simulink model "OSWT"  (R2022a)
settings: Solver=ode5  StartTime=0.0  StopTime=inf  RelTol=1e-3
model workspace (MAT data in the model file):
  autoELoad = 0
  autoPitch = 0
  eLoad = 0
  pitch = 0
libraries: simulink x1, sldrtlib x1
settings Model: SimulationMode=external  Creator=segu222  LastModifiedBy=belensanchezcenteno
settings DataIOCC: ReturnWorkspaceOutputs=off
settings DebuggingCC: UnconnectedInputMsg=warning  UnconnectedOutputMsg=warning  UnconnectedLineMsg=warning
settings HardwareCC: ProdBitPerLong=64  ProdHWDeviceType=Intel->x86-64 (Linux 64)
settings RTWCC: Description=Simulink Desktop Real-Time  SystemTargetFile=sldrt.tlc  TemplateMakefile=sldrt.tmf  RTWCompilerOptimization=on  DLArmComputeVersion=19.05
settings CodeAppCC: MaxIdLength=95
settings SimulinkDesktopRealTimeCC: TargetLibSuffix=_sldrt.a  TargetPreCompLibLocation=/Applications/MATLAB_R2022a.app/toolbox/sldrt/lib/maci64

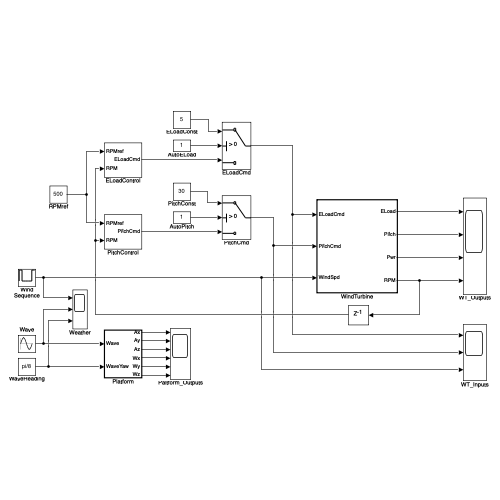
[thumbnail: Simulink's stored preview of the top-level diagram]
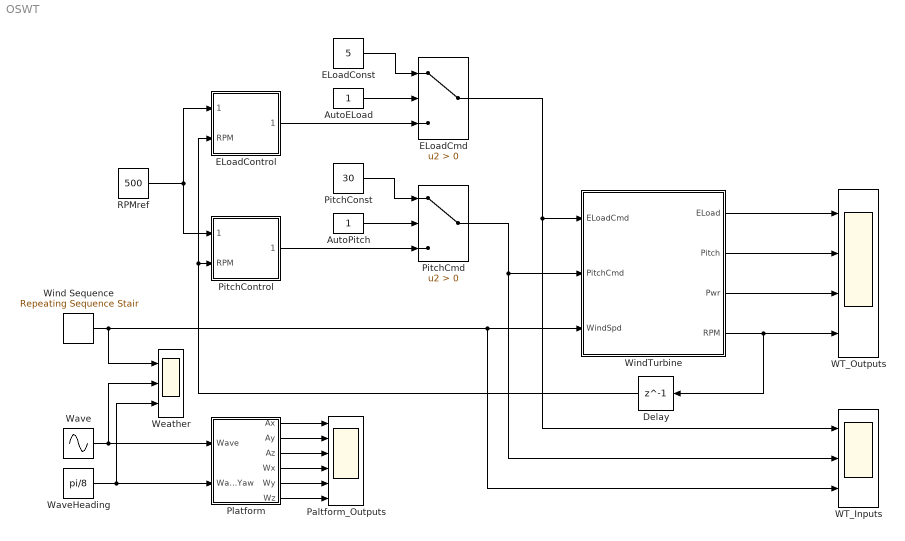
== system OSWT ==
  AutoELoad : Constant
  AutoPitch : Constant  VectorParams1D=off
  Delay : Delay  DelayLength=1
  ELoadCmd : Switch  Criteria=u2 > Threshold  SaturateOnIntegerOverflow=off  InputSameDT=off
  ELoadConst : Constant  Value=5
  ELoadControl : Subsystem
  Paltform_Outputs : Scope  NumInputPorts=6
  PitchCmd : Switch  Criteria=u2 > Threshold  SaturateOnIntegerOverflow=off  InputSameDT=off
  PitchConst : Constant  Value=30
  PitchControl : Subsystem
  Platform : Subsystem  TreatAsAtomicUnit=on
  RPMref : Constant  Value=500
  WT_Inputs : Scope  NumInputPorts=3
  WT_Outputs : Scope  NumInputPorts=4
  Wave : Sin  Frequency=2*pi/6  SampleTime=0
  WaveHeading : Constant  Value=pi/8
  Weather : Scope  NumInputPorts=3
  Wind Sequence : simulink/Sources/Repeating Sequence Stair  OutValues=[12 12 10 10 10 10 10 10 12 12]  tsamp=20  OutMin=[]  OutMax=[]  OutDataTypeStr=double  OutputDataTypeScalingMode=double  OutDataType=fixdt(0,8)  ConRadixGroup=Best Precision: Vector-wise  OutScaling=2^-12
  WindTurbine : Subsystem  TreatAsAtomicUnit=on
  wires:
  Wind Sequence/1 -> Weather/1, WT_Inputs/3, WindTurbine/3(WindSpd)
  ELoadCmd/1 -> WT_Inputs/1, WindTurbine/1(ELoadCmd)
  PitchCmd/1 -> WT_Inputs/2, WindTurbine/2(PitchCmd)
  RPMref/1 -> PitchControl/1(RPMref), ELoadControl/1(RPMref)
  WindTurbine/3(Pwr) -> WT_Outputs/3
  WindTurbine/2(Pitch) -> WT_Outputs/2
  WindTurbine/1(ELoad) -> WT_Outputs/1
  Wave/1 -> Weather/2, Platform/1(Wave)
  WaveHeading/1 -> Weather/3, Platform/2(WaveYaw)
  Platform/1(Ax) -> Paltform_Outputs/1
  Platform/2(Ay) -> Paltform_Outputs/2
  Platform/3(Az) -> Paltform_Outputs/3
  Platform/4(Wx) -> Paltform_Outputs/4
  Platform/5(Wy) -> Paltform_Outputs/5
  Platform/6(Wz) -> Paltform_Outputs/6
  WindTurbine/4(RPM) -> Delay/1, WT_Outputs/4
  AutoELoad/1 -> ELoadCmd/2
  AutoPitch/1 -> PitchCmd/2
  ELoadControl/1(ELoadCmd) -> ELoadCmd/3
  ELoadConst/1 -> ELoadCmd/1
  PitchControl/1(PitchCmd) -> PitchCmd/3
  PitchConst/1 -> PitchCmd/1
  Delay/1 -> ELoadControl/2(RPM), PitchControl/2(RPM)

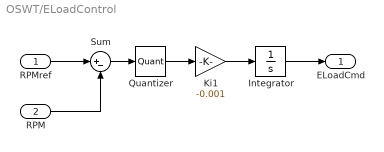
== system OSWT/ELoadControl ==
  RPMref : Inport
  RPM : Inport  Port=2
  Integrator : Integrator  LimitOutput=on  UpperSaturationLimit=15  LowerSaturationLimit=0
  Ki1 : Gain  Gain=-0.001
  Quantizer : Quantizer  QuantizationInterval=50
  Sum : Sum  Inputs=|+-
  ELoadCmd : Outport
  wires:
  RPMref/1 -> Sum/1
  Ki1/1 -> Integrator/1
  Sum/1 -> Quantizer/1
  Quantizer/1 -> Ki1/1
  Integrator/1 -> ELoadCmd/1
  RPM/1 -> Sum/2

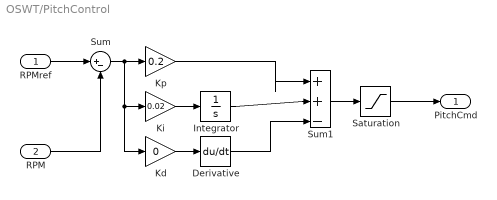
== system OSWT/PitchControl ==
  RPMref : Inport
  RPM : Inport  Port=2
  Derivative : Derivative
  Integrator : Integrator  InitialCondition=10  LimitOutput=on  UpperSaturationLimit=45  LowerSaturationLimit=-45
  Kd : Gain  Gain=0
  Ki : Gain  Gain=0.02
  Kp : Gain  Gain=0.2
  Saturation : Saturate  UpperLimit=45  LowerLimit=0
  Sum : Sum  Inputs=|+-
  Sum1 : Sum  Inputs=|++-
  PitchCmd : Outport
  wires:
  RPMref/1 -> Sum/1
  Sum/1 -> Kd/1, Ki/1, Kp/1
  Kp/1 -> Sum1/1
  RPM/1 -> Sum/2
  Ki/1 -> Integrator/1
  Integrator/1 -> Sum1/2
  Kd/1 -> Derivative/1
  Derivative/1 -> Sum1/3
  Sum1/1 -> Saturation/1
  Saturation/1 -> PitchCmd/1

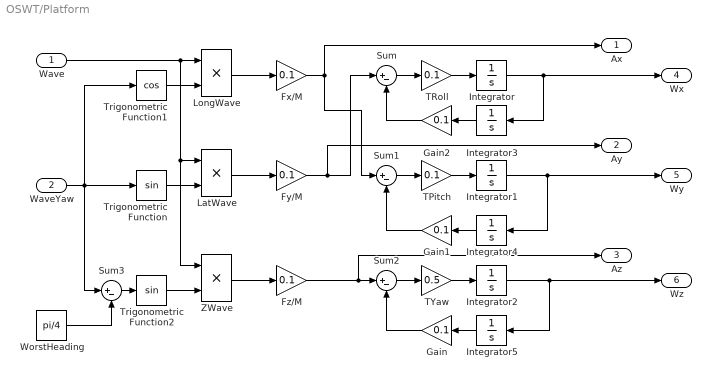
== system OSWT/Platform ==
  Wave : Inport
  WaveYaw : Inport  Port=2
  Fx/M : Gain  Gain=0.1
  Fy/M : Gain  Gain=0.1
  Fz/M : Gain  Gain=0.1
  Gain : Gain  Gain=0.1
  Gain1 : Gain  Gain=0.1
  Gain2 : Gain  Gain=0.1
  Integrator : Integrator  UpperSaturationLimit=1  LowerSaturationLimit=-45
  Integrator1 : Integrator  UpperSaturationLimit=1  LowerSaturationLimit=-45
  Integrator2 : Integrator  UpperSaturationLimit=1  LowerSaturationLimit=-45
  Integrator3 : Integrator
  Integrator4 : Integrator
  Integrator5 : Integrator
  LatWave : Product
  LongWave : Product
  Sum{,1..3} (4 alike) : Sum  Inputs=|+-
  TPitch : Gain  Gain=0.1
  TRoll : Gain  Gain=0.1
  TYaw : Gain  Gain=0.5
  Trigonometric Function : Trigonometry
  Trigonometric Function1 : Trigonometry  Operator=cos
  Trigonometric Function2 : Trigonometry
  WorstHeading : Constant  Value=pi/4
  ZWave : Product
  Ax : Outport
  Ay : Outport  Port=2
  Az : Outport  Port=3
  Wx : Outport  Port=4
  Wy : Outport  Port=5
  Wz : Outport  Port=6
  wires:
  WaveYaw/1 -> Sum3/1, Trigonometric Function1/1, Trigonometric Function/1
  Trigonometric Function/1 -> LatWave/2
  Trigonometric Function1/1 -> LongWave/2
  LongWave/1 -> Fx/M/1
  Fy/M/1 -> Sum/1, Ay/1
  Fz/M/1 -> Az/1, Sum2/1
  Integrator2/1 -> Integrator5/1, Wz/1
  TPitch/1 -> Integrator1/1
  TRoll/1 -> Integrator/1
  TYaw/1 -> Integrator2/1
  Integrator1/1 -> Integrator4/1, Wy/1
  Integrator/1 -> Integrator3/1, Wx/1
  Fx/M/1 -> Sum1/1, Ax/1
  LatWave/1 -> Fy/M/1
  Integrator3/1 -> Gain2/1
  Sum/1 -> TRoll/1
  Integrator4/1 -> Gain1/1
  Sum1/1 -> TPitch/1
  Sum2/1 -> TYaw/1
  Integrator5/1 -> Gain/1
  Gain/1 -> Sum2/2
  Gain1/1 -> Sum1/2
  Gain2/1 -> Sum/2
  Wave/1 -> LongWave/1, ZWave/1, LatWave/1
  WorstHeading/1 -> Sum3/2
  Sum3/1 -> Trigonometric Function2/1
  Trigonometric Function2/1 -> ZWave/2
  ZWave/1 -> Fz/M/1

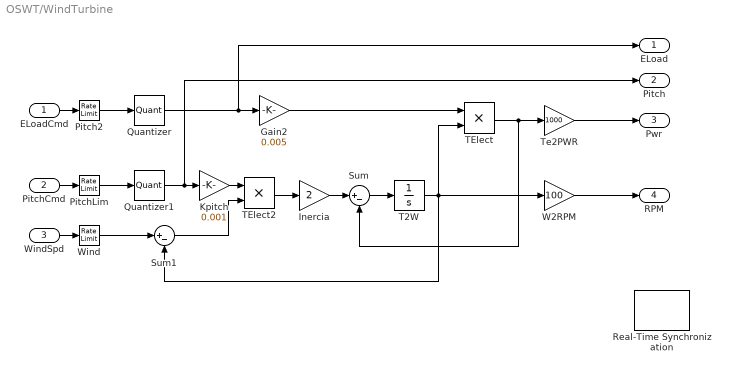
== system OSWT/WindTurbine ==
  ELoadCmd : Inport
  PitchCmd : Inport  Port=2
  WindSpd : Inport  Port=3
  Gain2 : Gain  Gain=0.005
  Inercia : Gain  Gain=2
  Kpitch : Gain  Gain=0.001
  Pitch2 : RateLimiter  RisingSlewLimit=0.2  FallingSlewLimit=-0.2
  PitchLim : RateLimiter  RisingSlewLimit=2  FallingSlewLimit=-2
  Quantizer : Quantizer  QuantizationInterval=1
  Quantizer1 : Quantizer  QuantizationInterval=1
  Real-Time Synchronization : sldrtlib/Real-Time Synchronization  SampleTime=0.1  MaxMissedTicks=10  ShowMissedTicks=off  YieldWhenWaiting=off
  Sum : Sum  Inputs=|+-
  Sum1 : Sum  Inputs=|+-
  T2W : Integrator
  TElect : Product
  TElect2 : Product
  Te2PWR : Gain  Gain=1000
  W2RPM : Gain  Gain=100
  Wind : RateLimiter
  ELoad : Outport
  Pitch : Outport  Port=2
  Pwr : Outport  Port=3
  RPM : Outport  Port=4
  wires:
  Gain2/1 -> TElect/1
  T2W/1 -> TElect/2, W2RPM/1, Sum1/2
  PitchLim/1 -> Quantizer1/1
  W2RPM/1 -> RPM/1
  Te2PWR/1 -> Pwr/1
  PitchCmd/1 -> PitchLim/1
  WindSpd/1 -> Wind/1
  TElect/1 -> Sum/2, Te2PWR/1
  Kpitch/1 -> TElect2/1
  ELoadCmd/1 -> Pitch2/1
  Pitch2/1 -> Quantizer/1
  Quantizer/1 -> ELoad/1, Gain2/1
  Wind/1 -> Sum1/1
  Sum1/1 -> TElect2/2
  TElect2/1 -> Inercia/1
  Sum/1 -> T2W/1
  Inercia/1 -> Sum/1
  Quantizer1/1 -> Pitch/1, Kpitch/1
